simulink subsystem "Unfinished_NLADRC"  (R2024b)
settings: Solver=VariableStepAuto  StartTime=0.0  StopTime=10.0  RelTol=1e-3
values from neighbouring files (symbols this model uses):
  A1 = 3.1416e-04    (= 0.00031416)    [InitialParameter.m]    (also in pneumatic_code.m = 0.000314159265359)
  A2 = 2.6389e-04    (= 0.00026389)    [InitialParameter.m]    (also in pneumatic_code.m = 0.000263893782902)
  b = 1    [InitialParameter.m]    (also in pneumatic_code.m = 0.0025)
  ep = 0.0024    [InitialParameter.m]    (also in pneumatic_code.m = 0.02)
  k = 1.4    [pneumatic_code.m]
  k1 = wc^4    (= 81450625)    [InitialParameter.m]    (also in pneumatic_code.m = 3620506.28125)
  k2 = 4*wc^3    (= 3429500)    [InitialParameter.m]    (also in pneumatic_code.m = 883050.3125)
  k3 = 6*wc^2    (= 54150)    [InitialParameter.m]    (also in pneumatic_code.m = 86151.25)
undefined symbols (not defined in the file or in its folder): bt, P1, P2, V1, V2
settings Model: Creator=pangl  LastModifiedBy=pangl

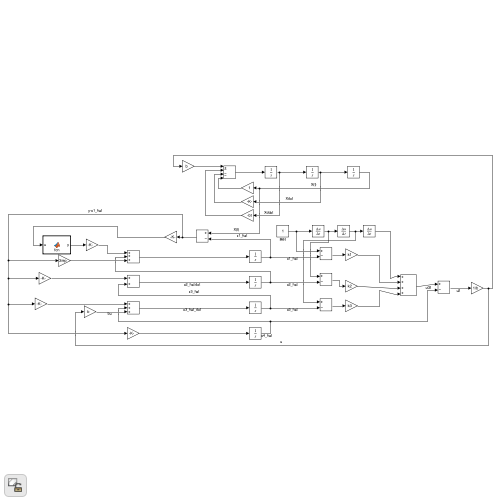
[thumbnail: Simulink's stored preview of the top-level diagram]
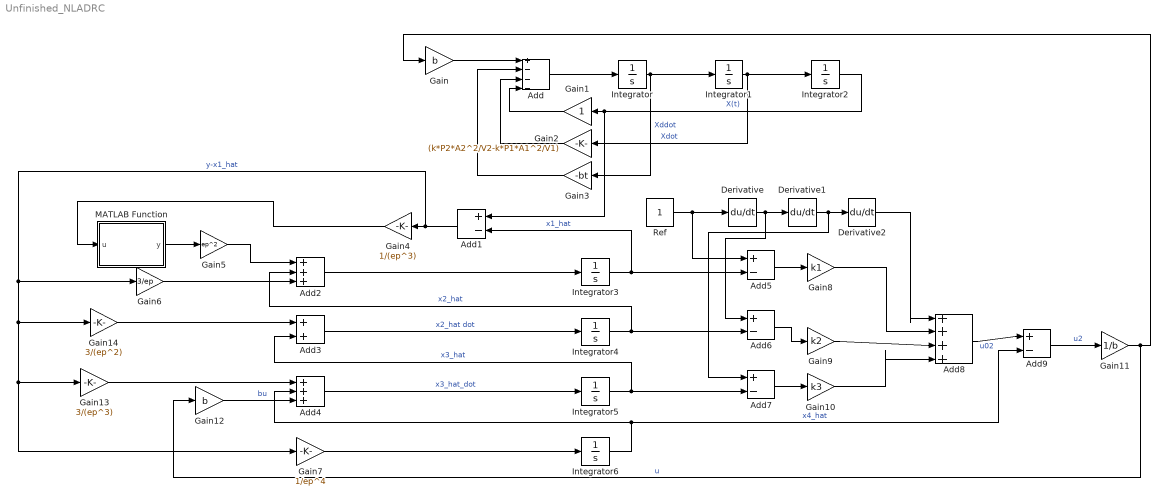
== system Unfinished_NLADRC ==
  Add : Sum  Inputs=+---
  Add{1,5..7,9} (5 alike) : Sum  Inputs=+-
  Add2 : Sum  Inputs=+++
  Add3 : Sum
  Add4 : Sum  Inputs=+++
  Add8 : Sum  Inputs=++++
  Derivative : Derivative
  Derivative1 : Derivative
  Derivative2 : Derivative
  Gain : Gain  Gain=b
  Gain1 : Gain
  Gain10 : Gain  Gain=k3
  Gain11 : Gain  Gain=1/b
  Gain12 : Gain  Gain=b
  Gain13 : Gain  Gain=3/(ep^3)
  Gain14 : Gain  Gain=3/(ep^2)
  Gain2 : Gain  Gain=(k*P2*A2^2/V2-k*P1*A1^2/V1)
  Gain3 : Gain  Gain=-bt
  Gain4 : Gain  Gain=1/(ep^3)
  Gain5 : Gain  Gain=ep^2
  Gain6 : Gain  Gain=3/ep
  Gain7 : Gain  Gain=1/ep^4
  Gain8 : Gain  Gain=k1
  Gain9 : Gain  Gain=k2
  Integrator{,1..6} (7 alike) : Integrator
  MATLAB Function : MATLAB Function  TreatAsAtomicUnit=on
  Ref : Constant
  wires:
  Add7/1 -> Gain10/1
  Derivative/1 -> Derivative1/1, Add6/1
  Gain9/1 -> Add8/3
  Gain6/1 -> Add2/3
  Add9/1 -> Gain11/1  "u2"
  Gain13/1 -> Add4/1
  Add6/1 -> Gain9/1
  Add2/1 -> Integrator3/1
  Gain12/1 -> Add4/3  "bu"
  Add8/1 -> Add9/1  "u02"
  Integrator1/1 -> Integrator2/1, Gain2/1  "Xdot"
  Gain5/1 -> Add2/1
  Gain8/1 -> Add8/2
  Gain14/1 -> Add3/1
  Gain4/1 -> MATLAB Function/1(u)
  Integrator4/1 -> Add2/2, Add6/2  "x2_hat"
  Integrator6/1 -> Add4/2, Add9/2  "x4_hat"
  Integrator/1 -> Integrator1/1, Gain3/1  "Xddot"
  Add3/1 -> Integrator4/1  "x2_hat dot"
  Gain1/1 -> Add/4
  Gain10/1 -> Add8/4
  Add1/1 -> Gain4/1, Gain13/1, Gain7/1, Gain14/1, Gain6/1  "y-x1_hat"
  Gain2/1 -> Add/3
  Gain7/1 -> Integrator6/1
  Ref/1 -> Derivative/1, Add5/1
  Gain3/1 -> Add/2
  MATLAB Function/1(y) -> Gain5/1
  Add5/1 -> Gain8/1
  Gain11/1 -> Gain/1, Gain12/1  "u"
  Add/1 -> Integrator/1
  Derivative2/1 -> Add8/1
  Derivative1/1 -> Derivative2/1, Add7/1
  Integrator2/1 -> Gain1/1, Add1/1  "X(t)"
  Integrator3/1 -> Add5/2, Add1/2  "x1_hat"
  Add4/1 -> Integrator5/1  "x3_hat_dot"
  Gain/1 -> Add/1
  Integrator5/1 -> Add3/2, Add7/2  "x3_hat"

== matlab function Unfinished_NLADRC/MATLAB Function ==
  data: u input; y output
function y = fcn(u)

if  u<= -pi/2
    y=-(1/4*pi);
elseif u< pi/2 && u> -pi/2
    y=sin(u)/(4*pi);
elseif u>pi/2
    y=1/(4*pi);
end
